simulink model "EjemploClaseSimulink"  (R2016a)
settings: Solver=VariableStepAuto  StartTime=0.0  StopTime=10  RelTol=1e-3
values from neighbouring files (symbols this model uses):
  A = [ 0 1 0 ; 0 0 1; -1 -5 -6]    [Guia_9_Ejercicio_2.m]
  B = [0; 0 ; 1]    [Guia_9_Ejercicio_2.m]
  C = KCRAF * KCRRF * GRRF * GRAF    [ejercicio5guia8.m]
undefined symbols (not defined in the file or in its folder): D
libraries: simulink x1
settings Model: Creator=Abel  LastModifiedBy=Abel

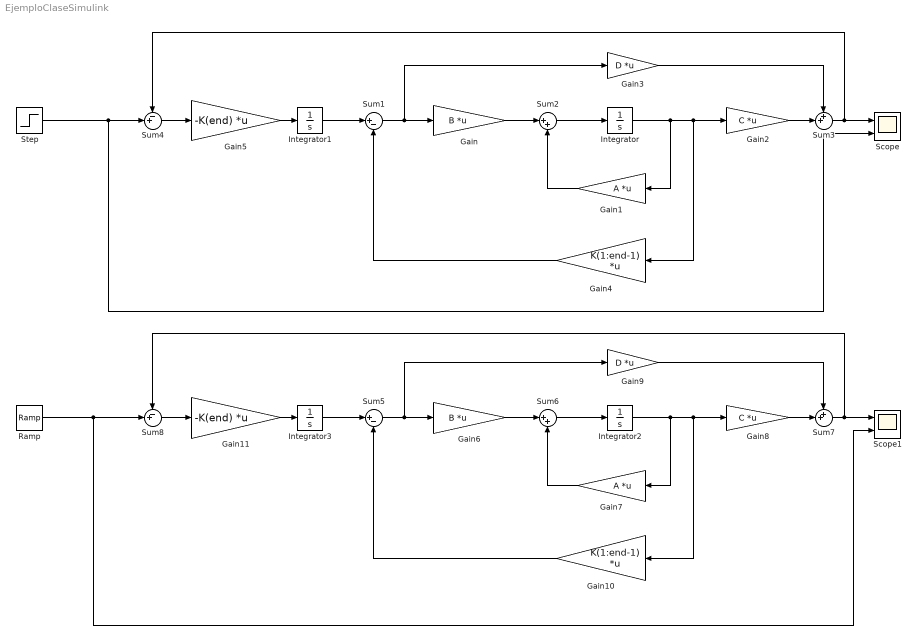
== system EjemploClaseSimulink ==
  Gain : Gain  Gain=B  Multiplication=Matrix(K*u) (u vector)
  Gain1 : Gain  Gain=A  Multiplication=Matrix(K*u) (u vector)
  Gain10 : Gain  Gain=K(1:end-1)  Multiplication=Matrix(K*u) (u vector)
  Gain11 : Gain  Gain=-K(end)  Multiplication=Matrix(K*u) (u vector)
  Gain2 : Gain  Gain=C  Multiplication=Matrix(K*u) (u vector)
  Gain3 : Gain  Gain=D  Multiplication=Matrix(K*u) (u vector)
  Gain4 : Gain  Gain=K(1:end-1)  Multiplication=Matrix(K*u) (u vector)
  Gain5 : Gain  Gain=-K(end)  Multiplication=Matrix(K*u) (u vector)
  Gain6 : Gain  Gain=B  Multiplication=Matrix(K*u) (u vector)
  Gain7 : Gain  Gain=A  Multiplication=Matrix(K*u) (u vector)
  Gain8 : Gain  Gain=C  Multiplication=Matrix(K*u) (u vector)
  Gain9 : Gain  Gain=D  Multiplication=Matrix(K*u) (u vector)
  Integrator{,1..3} (4 alike) : Integrator
  Ramp : simulink/Sources/Ramp  slope=1  start=0  X0=0
  Scope : Scope  NumInputPorts=2
  Scope1 : Scope  NumInputPorts=2
  Step : Step  SampleTime=0
  Sum1 : Sum  Inputs=|+-
  Sum2 : Sum  Inputs=|++
  Sum3 : Sum  Inputs=++|
  Sum4 : Sum  Inputs=-+|
  Sum5 : Sum  Inputs=|+-
  Sum6 : Sum  Inputs=|++
  Sum7 : Sum  Inputs=++|
  Sum8 : Sum  Inputs=-+|
  wires:
  Sum1/1 -> Gain3/1, Gain/1
  Gain/1 -> Sum2/1
  Sum2/1 -> Integrator/1
  Gain1/1 -> Sum2/2
  Integrator/1 -> Gain4/1, Gain2/1, Gain1/1
  Gain2/1 -> Sum3/2
  Gain3/1 -> Sum3/1
  Sum3/1 -> Scope/1, Sum4/1
  Gain4/1 -> Sum1/2
  Sum4/1 -> Gain5/1
  Step/1 -> Sum4/2, Scope/2
  Gain5/1 -> Integrator1/1
  Integrator1/1 -> Sum1/1
  Sum5/1 -> Gain9/1, Gain6/1
  Gain6/1 -> Sum6/1
  Sum6/1 -> Integrator2/1
  Gain7/1 -> Sum6/2
  Integrator2/1 -> Gain10/1, Gain8/1, Gain7/1
  Gain8/1 -> Sum7/2
  Gain9/1 -> Sum7/1
  Sum7/1 -> Scope1/1, Sum8/1
  Gain10/1 -> Sum5/2
  Sum8/1 -> Gain11/1
  Gain11/1 -> Integrator3/1
  Integrator3/1 -> Sum5/1
  Ramp/1 -> Sum8/2, Scope1/2
